simulink model "CrCtl_Governor"  (R2016b)
settings: configuration reference "CodeGenConfigSet" (kept outside this file)
values from neighbouring files (symbols this model uses):
  ACC_ZERO = fi(0,Acc_m_s2)    [init_CrCtl_Governor.m]
  CrCtl_facAcc2TrqCor_C = Calibration.Parameter    [init_CrCtl_Governor.m]
  CrCtl_facDecl2TrqCor_C = Calibration.Parameter    [init_CrCtl_Governor.m]
  CrCtl_facPT11_C = Calibration.Parameter    [init_CrCtl_Governor.m]
  CrCtl_facPT12_C = Calibration.Parameter    [init_CrCtl_Governor.m]
  CrCtl_facPT13_C = Calibration.Parameter    [init_CrCtl_Governor.m]
  CrCtl_facRmpSlpHiAcc_C = Calibration.Parameter    [init_CrCtl_Governor.m]
  CrCtl_facRmpSlpHiDecl_C = Calibration.Parameter    [init_CrCtl_Governor.m]
  CrCtl_facSlpConstRmpDwn_C = Calibration.Parameter    [init_CrCtl_Governor.m]
  CrCtl_facSlpConstRmpUp_C = Calibration.Parameter    [init_CrCtl_Governor.m]
  CrCtl_facSlpRmp1Sus_C = Calibration.Parameter    [init_CrCtl_Governor.m]
  CrCtl_facSlpRmp2Sus_C = Calibration.Parameter    [init_CrCtl_Governor.m]
  CrCtl_facTipDwnCor_CUR = Calibration.Parameter    [init_CrCtl_Governor.m]
  CrCtl_facTipDwnCor_CURX = Calibration.Parameter    [init_CrCtl_Governor.m]
  CrCtl_facTipUpCor_CUR = Calibration.Parameter    [init_CrCtl_Governor.m]
  CrCtl_facTipUpCor_CURX = Calibration.Parameter    [init_CrCtl_Governor.m]
  CrCtl_facTrqIncrSlpConstRmp_C = Calibration.Parameter    [init_CrCtl_Governor.m]
  CrCtl_facTrqIncrTimeConstRmp_C = Calibration.Parameter    [init_CrCtl_Governor.m]
  CrCtl_facTrqRedSlpConstRmp_C = Calibration.Parameter    [init_CrCtl_Governor.m]
  CrCtl_facTrqRedTimeConstRmp_C = Calibration.Parameter    [init_CrCtl_Governor.m]
  CrCtl_facTrqStrtAcc_C = Calibration.Parameter    [init_CrCtl_Governor.m]
  CrCtl_KiAcc1IWin_C = Calibration.Parameter    [init_CrCtl_Governor.m]
  CrCtl_KiAcc2IWin_C = Calibration.Parameter    [init_CrCtl_Governor.m]
  CrCtl_KiAcc3IWin_C = Calibration.Parameter    [init_CrCtl_Governor.m]
  CrCtl_KiCruise1IWin_C = Calibration.Parameter    [init_CrCtl_Governor.m]
  CrCtl_KiCruise2IWin_C = Calibration.Parameter    [init_CrCtl_Governor.m]
  CrCtl_KiCruise3IWin_C = Calibration.Parameter    [init_CrCtl_Governor.m]
  CrCtl_KiDecl1IWin_C = Calibration.Parameter    [init_CrCtl_Governor.m]
  CrCtl_KiDecl2IWin_C = Calibration.Parameter    [init_CrCtl_Governor.m]
  CrCtl_KiDecl3IWin_C = Calibration.Parameter    [init_CrCtl_Governor.m]
  CrCtl_KiNegAcc1IWin_C = Calibration.Parameter    [init_CrCtl_Governor.m]
  CrCtl_KiNegAcc2IWin_C = Calibration.Parameter    [init_CrCtl_Governor.m]
  CrCtl_KiNegAcc3IWin_C = Calibration.Parameter    [init_CrCtl_Governor.m]
  CrCtl_KiNegCruise1IWin_C = Calibration.Parameter    [init_CrCtl_Governor.m]
  CrCtl_KiNegCruise2IWin_C = Calibration.Parameter    [init_CrCtl_Governor.m]
  CrCtl_KiNegCruise3IWin_C = Calibration.Parameter    [init_CrCtl_Governor.m]
  CrCtl_KiNegDecl1IWin_C = Calibration.Parameter    [init_CrCtl_Governor.m]
  CrCtl_KiNegDecl2IWin_C = Calibration.Parameter    [init_CrCtl_Governor.m]
  CrCtl_KiNegDecl3IWin_C = Calibration.Parameter    [init_CrCtl_Governor.m]
  CrCtl_KiNegRes1IWin_C = Calibration.Parameter    [init_CrCtl_Governor.m]
  CrCtl_KiNegRes2IWin_C = Calibration.Parameter    [init_CrCtl_Governor.m]
  CrCtl_KiNegRes3IWin_C = Calibration.Parameter    [init_CrCtl_Governor.m]
  CrCtl_KiNegResCruise1IWin_C = Calibration.Parameter    [init_CrCtl_Governor.m]
  CrCtl_KiNegResCruise2IWin_C = Calibration.Parameter    [init_CrCtl_Governor.m]
  CrCtl_KiNegResCruise3IWin_C = Calibration.Parameter    [init_CrCtl_Governor.m]
  CrCtl_KiPosAcc1IWin_C = Calibration.Parameter    [init_CrCtl_Governor.m]
  CrCtl_KiPosAcc2IWin_C = Calibration.Parameter    [init_CrCtl_Governor.m]
  CrCtl_KiPosAcc3IWin_C = Calibration.Parameter    [init_CrCtl_Governor.m]
  CrCtl_KiPosCruise1IWin_C = Calibration.Parameter    [init_CrCtl_Governor.m]
  CrCtl_KiPosCruise2IWin_C = Calibration.Parameter    [init_CrCtl_Governor.m]
  CrCtl_KiPosCruise3IWin_C = Calibration.Parameter    [init_CrCtl_Governor.m]
  CrCtl_KiPosDecl1IWin_C = Calibration.Parameter    [init_CrCtl_Governor.m]
  CrCtl_KiPosDecl2IWin_C = Calibration.Parameter    [init_CrCtl_Governor.m]
  CrCtl_KiPosDecl3IWin_C = Calibration.Parameter    [init_CrCtl_Governor.m]
  CrCtl_KiPosRes1IWin_C = Calibration.Parameter    [init_CrCtl_Governor.m]
  CrCtl_KiPosRes3IWin_C = Calibration.Parameter    [init_CrCtl_Governor.m]
  CrCtl_KiPosResCruise1IWin_C = Calibration.Parameter    [init_CrCtl_Governor.m]
  CrCtl_KiPosResCruise2IWin_C = Calibration.Parameter    [init_CrCtl_Governor.m]
  CrCtl_KiPosResCruise3IWin_C = Calibration.Parameter    [init_CrCtl_Governor.m]
  CrCtl_KiRes1IWin_C = Calibration.Parameter    [init_CrCtl_Governor.m]
  CrCtl_KiRes2IWin_C = Calibration.Parameter    [init_CrCtl_Governor.m]
  CrCtl_KiRes3IWin_C = Calibration.Parameter    [init_CrCtl_Governor.m]
  CrCtl_KiResCruise1IWin_C = Calibration.Parameter    [init_CrCtl_Governor.m]
  CrCtl_KiResCruise2IWin_C = Calibration.Parameter    [init_CrCtl_Governor.m]
  CrCtl_KiResCruise3IWin_C = Calibration.Parameter    [init_CrCtl_Governor.m]
  CrCtl_KpAcc1PWin_C = Calibration.Parameter    [init_CrCtl_Governor.m]
  CrCtl_KpAcc2PWin_C = Calibration.Parameter    [init_CrCtl_Governor.m]
  CrCtl_KpAcc3PWin_C = Calibration.Parameter    [init_CrCtl_Governor.m]
  CrCtl_KpCruise1PWin_C = Calibration.Parameter    [init_CrCtl_Governor.m]
  CrCtl_KpCruise2PWin_C = Calibration.Parameter    [init_CrCtl_Governor.m]
  CrCtl_KpCruise3PWin_C = Calibration.Parameter    [init_CrCtl_Governor.m]
  CrCtl_KpDecl1PWin_C = Calibration.Parameter    [init_CrCtl_Governor.m]
  CrCtl_KpDecl2PWin_C = Calibration.Parameter    [init_CrCtl_Governor.m]
  CrCtl_KpDecl3PWin_C = Calibration.Parameter    [init_CrCtl_Governor.m]
  CrCtl_KpNegAcc1PWin_C = Calibration.Parameter    [init_CrCtl_Governor.m]
  CrCtl_KpNegAcc2PWin_C = Calibration.Parameter    [init_CrCtl_Governor.m]
  CrCtl_KpNegAcc3PWin_C = Calibration.Parameter    [init_CrCtl_Governor.m]
  CrCtl_KpNegCruise1PWin_C = Calibration.Parameter    [init_CrCtl_Governor.m]
  CrCtl_KpNegCruise2PWin_C = Calibration.Parameter    [init_CrCtl_Governor.m]
  CrCtl_KpNegCruise3PWin_C = Calibration.Parameter    [init_CrCtl_Governor.m]
  CrCtl_KpNegDecl1PWin_C = Calibration.Parameter    [init_CrCtl_Governor.m]
  CrCtl_KpNegDecl2PWin_C = Calibration.Parameter    [init_CrCtl_Governor.m]
  CrCtl_KpNegDecl3PWin_C = Calibration.Parameter    [init_CrCtl_Governor.m]
  CrCtl_KpNegRes1PWin_C = Calibration.Parameter    [init_CrCtl_Governor.m]
  CrCtl_KpNegRes2PWin_C = Calibration.Parameter    [init_CrCtl_Governor.m]
  CrCtl_KpNegRes3PWin_C = Calibration.Parameter    [init_CrCtl_Governor.m]
  CrCtl_KpNegResCruise1PWin_C = Calibration.Parameter    [init_CrCtl_Governor.m]
  CrCtl_KpNegResCruise2PWin_C = Calibration.Parameter    [init_CrCtl_Governor.m]
  CrCtl_KpNegResCruise3PWin_C = Calibration.Parameter    [init_CrCtl_Governor.m]
  CrCtl_KpPosAcc1PWin_C = Calibration.Parameter    [init_CrCtl_Governor.m]
  CrCtl_KpPosAcc2PWin_C = Calibration.Parameter    [init_CrCtl_Governor.m]
  CrCtl_KpPosAcc3PWin_C = Calibration.Parameter    [init_CrCtl_Governor.m]
  CrCtl_KpPosCruise1PWin_C = Calibration.Parameter    [init_CrCtl_Governor.m]
  CrCtl_KpPosCruise2PWin_C = Calibration.Parameter    [init_CrCtl_Governor.m]
  CrCtl_KpPosCruise3PWin_C = Calibration.Parameter    [init_CrCtl_Governor.m]
  CrCtl_KpPosDecl1PWin_C = Calibration.Parameter    [init_CrCtl_Governor.m]
  CrCtl_KpPosDecl2PWin_C = Calibration.Parameter    [init_CrCtl_Governor.m]
  CrCtl_KpPosDecl3PWin_C = Calibration.Parameter    [init_CrCtl_Governor.m]
  CrCtl_KpPosRes1PWin_C = Calibration.Parameter    [init_CrCtl_Governor.m]
  CrCtl_KpPosRes2PWin_C = Calibration.Parameter    [init_CrCtl_Governor.m]
  CrCtl_KpPosRes3PWin_C = Calibration.Parameter    [init_CrCtl_Governor.m]
  CrCtl_KpPosResCruise1PWin_C = Calibration.Parameter    [init_CrCtl_Governor.m]
  CrCtl_KpPosResCruise2PWin_C = Calibration.Parameter    [init_CrCtl_Governor.m]
  CrCtl_KpPosResCruise3PWin_C = Calibration.Parameter    [init_CrCtl_Governor.m]
  CrCtl_KpRes1PWin_C = Calibration.Parameter    [init_CrCtl_Governor.m]
  CrCtl_KpRes2PWin_C = Calibration.Parameter    [init_CrCtl_Governor.m]
  CrCtl_KpRes3PWin_C = Calibration.Parameter    [init_CrCtl_Governor.m]
  CrCtl_KpResCruise1PWin_C = Calibration.Parameter    [init_CrCtl_Governor.m]
  CrCtl_KpResCruise2PWin_C = Calibration.Parameter    [init_CrCtl_Governor.m]
  CrCtl_KpResCruise3PWin_C = Calibration.Parameter    [init_CrCtl_Governor.m]
  CrCtl_numParSelThres1_C = Calibration.Parameter    [init_CrCtl_Governor.m]
  CrCtl_numParSelThres2_C = Calibration.Parameter    [init_CrCtl_Governor.m]
  CrCtl_swtBrkMode_C = Calibration.Parameter    [init_CrCtl_Governor.m]
  CrCtl_swtILimWithP_C = Calibration.Parameter    [init_CrCtl_Governor.m]
  CrCtl_swtOvrRdeFrzInteg_C = Calibration.Parameter    [init_CrCtl_Governor.m]
  CrCtl_swtParSelHysBrk_C = Calibration.Parameter    [init_CrCtl_Governor.m]
  CrCtl_swtPT1EngBrk_C = Calibration.Parameter    [init_CrCtl_Governor.m]
  CrCtl_swtSusRmpInit_C = Calibration.Parameter    [init_CrCtl_Governor.m]
  CrCtl_swtSusRmpStp_C = Calibration.Parameter    [init_CrCtl_Governor.m]
  CrCtl_swtTipUpDwnGvnrStrtVal_C = Calibration.Parameter    [init_CrCtl_Governor.m]
  ... (+88 more)
undefined symbols (not defined in the file or in its folder): CrCtl_Governor_DT, CrCtl_stLck_conv, CrCtl_stOpFunc_conv, CrCtl_stShOff_conv, CrCtl_stSub_conv, CrCtl_stSuspRamp_conv, CruiseCtl_State_conv, EBrk_stPreSelMode_conv, WESDem_State_conv
libraries: CXLib x126, simulink x25
(part 5 of 6)

== system CrCtl_Governor/Resume From Below/CRCTL_SUBRMP/Governor ==
  CrCtl_trqLimAct : Inport
  CrCtl_trqMin : Inport  Port=2
  CrCtl_stGearRng_mp : Inport  Port=3
  CrCtl_vDesAct : Inport  Port=4
  stvHysEngBrkReq : Inport  Port=5
  GlbDa_vXFlt : Inport  Port=6
  stCrCtlOn : Inport  Port=7
  In1 : Inport  Port=8
  In2 : Inport  Port=9
  Enable : EnablePort
  Add1 : Sum  Inputs=+-
  Add2 : Sum  OutDataTypeStr=Trq_Nm
  Add3 : Sum  OutDataTypeStr=Trq_Nm
  Constant : Constant  Value=CrCtl_swtILimWithP_C
  Constant1 : Constant  Value=CrCtl_Governor_DT
  Constant2 : Constant  Value=1000  OutDataTypeStr=Inherit: Inherit via back propagation
  CrCtl_ARW : Subsystem
  I_S16 : CXLib/I_S16
  PT1 Filtered Torque : Subsystem
  P_S16 : CXLib/P_S16
  Parameter Selection for Ki : Subsystem
  Parameter Selection for Kp : Subsystem
  Product : Product  OutDataTypeStr=uint32
  Saturation_S16 : CXLib/Saturation_S16
  Switch : Switch  Criteria=u2 ~= 0
  Terminator : Terminator
  Unit Delay : UnitDelay  SampleTime=-1
  Unit Delay1 : UnitDelay  SampleTime=-1
  CrCtl_trqReq : Outport
  CrCtl_trqIWinOld_mp : Outport  Port=2  OutDataTypeStr=Trq_Nm
  CrCtl_trqReqPWin_mp : Outport  Port=3
  wires:
  CrCtl_vDesAct/1 -> Add1/1
  GlbDa_vXFlt/1 -> Add1/2
  Add1/1 -> PT1 Filtered Torque/2(vDiffCrCtl), I_S16/1, P_S16/1
  Add2/1 -> Add3/1
  PT1 Filtered Torque/1(CrCtl_trqDesvHys) -> Add3/2
  Add3/1 -> Saturation_S16/1
  CrCtl_trqMin/1 -> CrCtl_ARW/2(CrCtl_trqMin), Saturation_S16/2
  CrCtl_trqLimAct/1 -> CrCtl_ARW/3(CrCtl_trqLimAct), Saturation_S16/3
  Saturation_S16/2 -> Terminator/1
  Saturation_S16/1 -> CrCtl_trqReq/1
  Switch/1 -> Add2/2, CrCtl_trqIWinOld_mp/1, CrCtl_ARW/5(CrCtl_trqReqIWin_mp)
  Constant/1 -> CrCtl_ARW/1(CrCtl_swtILimWithP_C)
  stvHysEngBrkReq/1 -> PT1 Filtered Torque/1(stvHysEngBrkReq)
  CrCtl_stGearRng_mp/1 -> Parameter Selection for Kp/1(CrCtl_stGearRng_mp), Parameter Selection for Ki/1(CrCtl_stGearRng_mp), PT1 Filtered Torque/3(CrCtl_stGearRng_mp)
  stCrCtlOn/1 -> PT1 Filtered Torque/4(stCrCtlOn)
  Parameter Selection for Kp/1(Out1) -> P_S16/2
  Parameter Selection for Kp/2(Out2) -> P_S16/3
  Parameter Selection for Kp/3(Out3) -> P_S16/4
  Parameter Selection for Kp/4(Out4) -> P_S16/5
  Parameter Selection for Kp/5(Out5) -> P_S16/6
  Parameter Selection for Ki/1(Out1) -> I_S16/3
  Parameter Selection for Ki/2(Out2) -> I_S16/4
  Parameter Selection for Ki/3(Out3) -> I_S16/5
  Parameter Selection for Ki/4(Out4) -> I_S16/6
  Parameter Selection for Ki/5(Out5) -> I_S16/7
  CrCtl_ARW/2(Limit) -> Unit Delay1/1
  CrCtl_ARW/1(CrCtl_stInit_mp) -> Unit Delay/1
  Product/1 -> I_S16/2
  Constant2/1 -> Product/2
  Constant1/1 -> Product/1
  P_S16/1 -> CrCtl_trqReqPWin_mp/1, CrCtl_ARW/4(CrCtl_trqReqPWin_mp), Add2/1
  In1/1 -> I_S16/8
  In2/1 -> I_S16/9
  I_S16/1 -> Switch/3
  Unit Delay/1 -> Switch/2
  Unit Delay1/1 -> Switch/1

== system CrCtl_Governor/Resume From Below/CRCTL_SUBSTRTVAL/Parameter Selection for Kp ==
  CrCtl_stGearRng_mp : Inport
  Constant1 : Constant  Value=CrCtl_KpRes2PWin_C
  Constant10 : Constant  Value=CrCtl_WinPosRes1PWin_C
  Constant11 : Constant  Value=CrCtl_WinPosRes2PWin_C
  Constant12 : Constant  Value=CrCtl_WinPosRes3PWin_C
  Constant13 : Constant  Value=CrCtl_WinNegRes1PWin_C
  Constant14 : Constant  Value=CrCtl_WinNegRes2PWin_C
  Constant15 : Constant  Value=CrCtl_WinNegRes3PWin_C
  Constant2 : Constant  Value=CrCtl_KpRes3PWin_C
  Constant3 : Constant  Value=CrCtl_KpPosRes1PWin_C
  Constant4 : Constant  Value=CrCtl_KpRes1PWin_C
  Constant5 : Constant  Value=CrCtl_KpPosRes2PWin_C
  Constant6 : Constant  Value=CrCtl_KpPosRes3PWin_C
  Constant7 : Constant  Value=CrCtl_KpNegRes1PWin_C
  Constant8 : Constant  Value=CrCtl_KpNegRes2PWin_C
  Constant9 : Constant  Value=CrCtl_KpNegRes3PWin_C
  Multiport Switch{,1..4} (5 alike) : MultiPortSwitch
  Out1 : Outport
  Out2 : Outport  Port=2
  Out3 : Outport  Port=3
  Out4 : Outport  Port=4
  Out5 : Outport  Port=5
  wires:
  CrCtl_stGearRng_mp/1 -> Multiport Switch4/1, Multiport Switch3/1, Multiport Switch2/1, Multiport Switch1/1, Multiport Switch/1
  Constant4/1 -> Multiport Switch/2
  Constant1/1 -> Multiport Switch/3
  Constant2/1 -> Multiport Switch/4
  Multiport Switch/1 -> Out1/1
  Constant3/1 -> Multiport Switch1/2
  Constant6/1 -> Multiport Switch1/4
  Constant5/1 -> Multiport Switch1/3
  Multiport Switch1/1 -> Out2/1
  Constant7/1 -> Multiport Switch2/2
  Constant9/1 -> Multiport Switch2/4
  Constant8/1 -> Multiport Switch2/3
  Constant10/1 -> Multiport Switch3/2
  Constant12/1 -> Multiport Switch3/4
  Constant11/1 -> Multiport Switch3/3
  Constant13/1 -> Multiport Switch4/2
  Constant15/1 -> Multiport Switch4/4
  Constant14/1 -> Multiport Switch4/3
  Multiport Switch2/1 -> Out3/1
  Multiport Switch3/1 -> Out4/1
  Multiport Switch4/1 -> Out5/1

== system CrCtl_Governor/Tip Down State/CRCTL_SUBCALCSET /Parameter Selection for Kp ==
  CrCtl_stGearRng_mp : Inport
  Constant1 : Constant  Value=CrCtl_KpDecl2PWin_C
  Constant10 : Constant  Value=CrCtl_WinPosDecl1PWin_C
  Constant11 : Constant  Value=CrCtl_WinPosDecl2PWin_C
  Constant12 : Constant  Value=CrCtl_WinPosDecl3PWin_C
  Constant13 : Constant  Value=CrCtl_WinNegDecl1PWin_C
  Constant14 : Constant  Value=CrCtl_WinNegDecl2PWin_C
  Constant15 : Constant  Value=CrCtl_WinNegDecl3PWin_C
  Constant2 : Constant  Value=CrCtl_KpDecl3PWin_C
  Constant3 : Constant  Value=CrCtl_KpPosDecl1PWin_C
  Constant4 : Constant  Value=CrCtl_KpDecl1PWin_C
  Constant5 : Constant  Value=CrCtl_KpPosDecl2PWin_C
  Constant6 : Constant  Value=CrCtl_KpPosDecl3PWin_C
  Constant7 : Constant  Value=CrCtl_KpNegDecl1PWin_C
  Constant8 : Constant  Value=CrCtl_KpNegDecl2PWin_C
  Constant9 : Constant  Value=CrCtl_KpNegDecl3PWin_C
  Multiport Switch{,1..4} (5 alike) : MultiPortSwitch
  Out1 : Outport
  Out2 : Outport  Port=2
  Out3 : Outport  Port=3
  Out4 : Outport  Port=4
  Out5 : Outport  Port=5
  wires:
  CrCtl_stGearRng_mp/1 -> Multiport Switch4/1, Multiport Switch3/1, Multiport Switch2/1, Multiport Switch1/1, Multiport Switch/1
  Constant4/1 -> Multiport Switch/2
  Constant1/1 -> Multiport Switch/3
  Constant2/1 -> Multiport Switch/4
  Multiport Switch/1 -> Out1/1
  Constant3/1 -> Multiport Switch1/2
  Constant6/1 -> Multiport Switch1/4
  Constant5/1 -> Multiport Switch1/3
  Multiport Switch1/1 -> Out2/1
  Constant7/1 -> Multiport Switch2/2
  Constant9/1 -> Multiport Switch2/4
  Constant8/1 -> Multiport Switch2/3
  Constant10/1 -> Multiport Switch3/2
  Constant12/1 -> Multiport Switch3/4
  Constant11/1 -> Multiport Switch3/3
  Constant13/1 -> Multiport Switch4/2
  Constant15/1 -> Multiport Switch4/4
  Constant14/1 -> Multiport Switch4/3
  Multiport Switch2/1 -> Out3/1
  Multiport Switch3/1 -> Out4/1
  Multiport Switch4/1 -> Out5/1

== system CrCtl_Governor/Tip Up State/Subsystem/Parameter Selection for Kp ==
  CrCtl_stGearRng_mp : Inport
  Constant1 : Constant  Value=CrCtl_KpAcc2PWin_C
  Constant10 : Constant  Value=CrCtl_WinPosAcc1PWin_C
  Constant11 : Constant  Value=CrCtl_WinPosAcc2PWin_C
  Constant12 : Constant  Value=CrCtl_WinPosAcc3PWin_C
  Constant13 : Constant  Value=CrCtl_WinNegAcc1PWin_C
  Constant14 : Constant  Value=CrCtl_WinNegAcc2PWin_C
  Constant15 : Constant  Value=CrCtl_WinNegAcc3PWin_C
  Constant2 : Constant  Value=CrCtl_KpAcc3PWin_C
  Constant3 : Constant  Value=CrCtl_KpPosAcc1PWin_C
  Constant4 : Constant  Value=CrCtl_KpAcc1PWin_C
  Constant5 : Constant  Value=CrCtl_KpPosAcc2PWin_C
  Constant6 : Constant  Value=CrCtl_KpPosAcc3PWin_C
  Constant7 : Constant  Value=CrCtl_KpNegAcc1PWin_C
  Constant8 : Constant  Value=CrCtl_KpNegAcc2PWin_C
  Constant9 : Constant  Value=CrCtl_KpNegAcc3PWin_C
  Multiport Switch{,1..4} (5 alike) : MultiPortSwitch
  Out1 : Outport
  Out2 : Outport  Port=2
  Out3 : Outport  Port=3
  Out4 : Outport  Port=4
  Out5 : Outport  Port=5
  wires:
  CrCtl_stGearRng_mp/1 -> Multiport Switch4/1, Multiport Switch3/1, Multiport Switch2/1, Multiport Switch1/1, Multiport Switch/1
  Constant4/1 -> Multiport Switch/2
  Constant1/1 -> Multiport Switch/3
  Constant2/1 -> Multiport Switch/4
  Multiport Switch/1 -> Out1/1
  Constant3/1 -> Multiport Switch1/2
  Constant6/1 -> Multiport Switch1/4
  Constant5/1 -> Multiport Switch1/3
  Multiport Switch1/1 -> Out2/1
  Constant7/1 -> Multiport Switch2/2
  Constant9/1 -> Multiport Switch2/4
  Constant8/1 -> Multiport Switch2/3
  Constant10/1 -> Multiport Switch3/2
  Constant12/1 -> Multiport Switch3/4
  Constant11/1 -> Multiport Switch3/3
  Constant13/1 -> Multiport Switch4/2
  Constant15/1 -> Multiport Switch4/4
  Constant14/1 -> Multiport Switch4/3
  Multiport Switch2/1 -> Out3/1
  Multiport Switch3/1 -> Out4/1
  Multiport Switch4/1 -> Out5/1

== system CrCtl_Governor/Acceleration State/CRCTL_SUBRMP/CrCtl_Suspend/Subsystem ==
  PT_trqWhlMinEng : Inport
  CrCtl_trqReqOld : Inport  Port=2
  CrCtl_stSuspAct : Inport  Port=3
  Enable : EnablePort
  Constant5 : Constant  Value=CrCtl_swtSusRmpStp_C
  Constant7 : Constant  Value=CrCtl_facSlpRmp1Sus_C
  Constant8 : Constant  Value=CrCtl_Governor_DT
  RAMP_S16 : CXLib/RAMP_S16
  Relational Operator : RelationalOperator  Operator=~=  OutDataTypeStr=boolean  RndMeth=Simplest
  Switch3 : Switch  Criteria=u2 ~= 0
  s2dt : CXLib/s2dt
  Out : Outport
  Out1 : Outport  Port=2
  wires:
  Constant7/1 -> s2dt/1
  Constant8/1 -> s2dt/2
  s2dt/1 -> RAMP_S16/3, RAMP_S16/2
  CrCtl_stSuspAct/1 -> RAMP_S16/4
  PT_trqWhlMinEng/1 -> Relational Operator/1, Switch3/1, RAMP_S16/1
  Relational Operator/1 -> Out/1
  CrCtl_trqReqOld/1 -> RAMP_S16/5
  Constant5/1 -> Switch3/2
  Switch3/1 -> Relational Operator/2, Out1/1
  RAMP_S16/1 -> Switch3/3

== system CrCtl_Governor/Acceleration State/CRCTL_SUBRMP/CrCtl_Suspend/Subsystem1 ==
  PT_trqWhlMinEng : Inport
  CrCtl_trqReqOld : Inport  Port=2
  AccPed_trqDes : Inport  Port=3
  CrCtl_trqLimAct : Inport  Port=4
  In1 : Inport  Port=5
  In2 : Inport  Port=6
  In3 : Inport  Port=7
  Enable : EnablePort
  Constant10 : Constant  Value=CrCtl_Governor_DT
  Constant6 : Constant  Value=CrCtl_swtSusRmpInit_C
  Constant9 : Constant  Value=CrCtl_facSlpRmp2Sus_C
  MinMax : MinMax  Function=max  Inputs=2
  MinMax1 : MinMax  Function=max  Inputs=2
  RAMP_S1 : CXLib/RAMP_S16
  Relational Operator1 : RelationalOperator  Operator=~=  OutDataTypeStr=boolean  RndMeth=Simplest
  Relational Operator2 : RelationalOperator  Operator=<  OutDataTypeStr=boolean  RndMeth=Simplest
  Relational Operator3 : RelationalOperator  Operator=<  OutDataTypeStr=boolean  RndMeth=Simplest
  Relational Operator4 : RelationalOperator  Operator=<  OutDataTypeStr=boolean  RndMeth=Simplest
  Switch{1..4,6} (5 alike) : Switch  Criteria=u2 ~= 0
  s2dt1 : CXLib/s2dt
  Out1 : Outport
  Out2 : Outport  Port=2
  wires:
  Constant9/1 -> s2dt1/1
  Constant10/1 -> s2dt1/2
  s2dt1/1 -> RAMP_S1/3, RAMP_S1/2
  CrCtl_trqReqOld/1 -> RAMP_S1/1, Relational Operator4/1, Switch6/1, MinMax/1, Relational Operator1/2, Switch2/1, Relational Operator3/1
  Constant6/1 -> Switch3/2
  MinMax/1 -> MinMax1/1
  MinMax1/1 -> Switch4/1, Relational Operator2/1
  CrCtl_trqLimAct/1 -> Switch4/3, Relational Operator2/2
  Relational Operator2/1 -> Switch4/2
  Switch4/1 -> Switch3/1
  AccPed_trqDes/1 -> Relational Operator3/2, MinMax1/2
  PT_trqWhlMinEng/1 -> Switch1/1, Relational Operator4/2, MinMax/2
  Relational Operator4/1 -> Switch1/2
  Switch3/1 -> Switch1/3
  Switch1/1 -> RAMP_S1/5
  In3/1 -> RAMP_S1/4
  In1/1 -> Switch6/2
  In2/1 -> Switch6/3
  Switch6/1 -> Switch3/3
  Relational Operator3/1 -> Switch2/2
  RAMP_S1/1 -> Switch2/3
  Switch2/1 -> Out2/1, Relational Operator1/1
  Relational Operator1/1 -> Out1/1

== system CrCtl_Governor/Acceleration State/CRCTL_SUBRMP/Governor/CrCtl_ARW ==
  CrCtl_swtILimWithP_C : Inport
  CrCtl_trqMin : Inport  Port=2
  CrCtl_trqLimAct : Inport  Port=3
  CrCtl_trqReqPWin_mp : Inport  Port=4
  CrCtl_trqReqIWin_mp : Inport  Port=5
  Add : Sum  Inputs=+-  OutDataTypeStr=Trq_Nm
  Add1 : Sum  Inputs=+-  OutDataTypeStr=Trq_Nm
  Relational Operator : RelationalOperator  Operator=<  OutDataTypeStr=boolean  RndMeth=Simplest
  Relational Operator1 : RelationalOperator  Operator=>  OutDataTypeStr=boolean  RndMeth=Simplest
  Saturation_S1 : CXLib/Saturation_S16
  Saturation_S16 : CXLib/Saturation_S16
  Switch{,1..3} (4 alike) : Switch  Criteria=u2 ~= 0
  CrCtl_stInit_mp : Outport
  Limit : Outport  Port=2
  wires:
  CrCtl_trqMin/1 -> Switch2/3, Relational Operator/2, Add/1, Saturation_S16/2
  CrCtl_trqLimAct/1 -> Switch3/3, Relational Operator1/2, Add1/1, Saturation_S16/3
  CrCtl_trqReqIWin_mp/1 -> Relational Operator1/1, Relational Operator/1, Saturation_S1/1, Saturation_S16/1
  CrCtl_swtILimWithP_C/1 -> Switch1/2, Switch/2
  Switch/1 -> CrCtl_stInit_mp/1
  Saturation_S16/2 -> Switch/3
  CrCtl_trqReqPWin_mp/1 -> Add1/2, Add/2
  Saturation_S1/2 -> Switch/1
  Saturation_S1/1 -> Switch1/1
  Saturation_S16/1 -> Switch1/3
  Switch1/1 -> Limit/1
  Switch2/1 -> Saturation_S1/2
  Switch3/1 -> Saturation_S1/3
  Add/1 -> Switch2/1
  Add1/1 -> Switch3/1
  Relational Operator/1 -> Switch2/2
  Relational Operator1/1 -> Switch3/2

== system CrCtl_Governor/Acceleration State/CRCTL_SUBRMP/Governor/PT1 Filtered Torque ==
  stvHysEngBrkReq : Inport
  vDiffCrCtl : Inport  Port=2
  CrCtl_stGearRng_mp : Inport  Port=3
  stCrCtlOn : Inport  Port=4
  Add : Sum  Inputs=+-
  Constant : Constant
  Constant1 : Constant  Value=CrCtl_swtPT1EngBrk_C
  Constant2 : Constant  Value=CrCtl_vEngBrkOffChkOfs_C
  Constant3 : Constant  Value=CrCtl_vHysEngBrkMode_C
  Constant4 : Constant  Value=0.0  OutDataTypeStr=Inherit: Inherit via back propagation
  Constant5 : Constant  Value=0  OutDataTypeStr=VehSpeed_km_h
  Logical Operator : Logic  Operator=NOT  AllPortsSameDT=off  OutDataTypeStr=boolean
  Logical Operator1 : Logic  Operator=OR  AllPortsSameDT=off  OutDataTypeStr=boolean
  PT1_S16 : CXLib/PT1_S16
  Parameter selection of PT1 : Subsystem
  Product : Product  OutDataTypeStr=Trq_Nm
  Relational Operator : RelationalOperator  Operator===  OutDataTypeStr=boolean  RndMeth=Simplest
  Switch : Switch  Criteria=u2 ~= 0
  Switch1 : Switch  Criteria=u2 ~= 0
  Switch2 : Switch  Criteria=u2 ~= 0
  CrCtl_trqDesvHys : Outport
  wires:
  Constant1/1 -> Relational Operator/1
  Constant/1 -> Relational Operator/2
  stvHysEngBrkReq/1 -> Logical Operator/1
  Relational Operator/1 -> Logical Operator1/1
  Logical Operator/1 -> Logical Operator1/2
  Constant2/1 -> Add/1
  Constant3/1 -> Add/2
  Logical Operator1/1 -> Switch1/2, Switch/2
  Add/1 -> Switch/3
  vDiffCrCtl/1 -> Switch/1
  CrCtl_stGearRng_mp/1 -> Parameter selection of PT1/1(CrCtl_stGearRng_mp)
  Parameter selection of PT1/1(Out1) -> PT1_S16/1
  Product/1 -> PT1_S16/2
  Parameter selection of PT1/2(Out2) -> Product/1
  PT1_S16/1 -> Switch1/1
  Constant4/1 -> Switch1/3
  Switch1/1 -> CrCtl_trqDesvHys/1  "CrCtl_trqPT1_mp"
  stCrCtlOn/1 -> Switch2/2
  Switch/1 -> Switch2/1
  Constant5/1 -> Switch2/3
  Switch2/1 -> Product/2

== system CrCtl_Governor/Acceleration State/CRCTL_SUBRMP/Governor/Parameter Selection for Ki ==
  CrCtl_stGearRng_mp : Inport
  Constant1 : Constant  Value=CrCtl_KiAcc2IWin_C
  Constant10 : Constant  Value=CrCtl_WinPosAcc1IWin_C
  Constant11 : Constant  Value=CrCtl_WinPosAcc2IWin_C
  Constant12 : Constant  Value=CrCtl_WinPosAcc3IWin_C
  Constant13 : Constant  Value=CrCtl_WinNegAcc1IWin_C
  Constant14 : Constant  Value=CrCtl_WinNegAcc2IWin_C
  Constant15 : Constant  Value=CrCtl_WinNegAcc3IWin_C
  Constant2 : Constant  Value=CrCtl_KiAcc3IWin_C
  Constant3 : Constant  Value=CrCtl_KiPosAcc1IWin_C
  Constant4 : Constant  Value=CrCtl_KiAcc1IWin_C
  Constant5 : Constant  Value=CrCtl_KiPosAcc2IWin_C
  Constant6 : Constant  Value=CrCtl_KiPosAcc3IWin_C
  Constant7 : Constant  Value=CrCtl_KiNegAcc1IWin_C
  Constant8 : Constant  Value=CrCtl_KiNegAcc2IWin_C
  Constant9 : Constant  Value=CrCtl_KiNegAcc3IWin_C
  Multiport Switch{,1..4} (5 alike) : MultiPortSwitch
  Out1 : Outport
  Out2 : Outport  Port=2
  Out3 : Outport  Port=3
  Out4 : Outport  Port=4
  Out5 : Outport  Port=5
  wires:
  Multiport Switch4/1 -> Out5/1
  Multiport Switch3/1 -> Out4/1
  Multiport Switch2/1 -> Out3/1
  Constant14/1 -> Multiport Switch4/3
  Constant15/1 -> Multiport Switch4/4
  Constant13/1 -> Multiport Switch4/2
  Constant11/1 -> Multiport Switch3/3
  Constant12/1 -> Multiport Switch3/4
  Constant10/1 -> Multiport Switch3/2
  Constant8/1 -> Multiport Switch2/3
  Constant9/1 -> Multiport Switch2/4
  Constant7/1 -> Multiport Switch2/2
  Multiport Switch1/1 -> Out2/1
  Constant5/1 -> Multiport Switch1/3
  Constant6/1 -> Multiport Switch1/4
  Constant3/1 -> Multiport Switch1/2
  Multiport Switch/1 -> Out1/1
  Constant2/1 -> Multiport Switch/4
  Constant1/1 -> Multiport Switch/3
  Constant4/1 -> Multiport Switch/2
  CrCtl_stGearRng_mp/1 -> Multiport Switch/1, Multiport Switch1/1, Multiport Switch2/1, Multiport Switch3/1, Multiport Switch4/1

== system CrCtl_Governor/Acceleration State/CRCTL_SUBRMP/Governor/Parameter Selection for Kp ==
  CrCtl_stGearRng_mp : Inport
  Constant1 : Constant  Value=CrCtl_KpAcc2PWin_C
  Constant10 : Constant  Value=CrCtl_WinPosAcc1PWin_C
  Constant11 : Constant  Value=CrCtl_WinPosAcc2PWin_C
  Constant12 : Constant  Value=CrCtl_WinPosAcc3PWin_C
  Constant13 : Constant  Value=CrCtl_WinNegAcc1PWin_C
  Constant14 : Constant  Value=CrCtl_WinNegAcc2PWin_C
  Constant15 : Constant  Value=CrCtl_WinNegAcc3PWin_C
  Constant2 : Constant  Value=CrCtl_KpAcc3PWin_C
  Constant3 : Constant  Value=CrCtl_KpPosAcc1PWin_C
  Constant4 : Constant  Value=CrCtl_KpAcc1PWin_C
  Constant5 : Constant  Value=CrCtl_KpPosAcc2PWin_C
  Constant6 : Constant  Value=CrCtl_KpPosAcc3PWin_C
  Constant7 : Constant  Value=CrCtl_KpNegAcc1PWin_C
  Constant8 : Constant  Value=CrCtl_KpNegAcc2PWin_C
  Constant9 : Constant  Value=CrCtl_KpNegAcc3PWin_C
  Multiport Switch{,1..4} (5 alike) : MultiPortSwitch
  Out1 : Outport
  Out2 : Outport  Port=2
  Out3 : Outport  Port=3
  Out4 : Outport  Port=4
  Out5 : Outport  Port=5
  wires:
  CrCtl_stGearRng_mp/1 -> Multiport Switch4/1, Multiport Switch3/1, Multiport Switch2/1, Multiport Switch1/1, Multiport Switch/1
  Constant4/1 -> Multiport Switch/2
  Constant1/1 -> Multiport Switch/3
  Constant2/1 -> Multiport Switch/4
  Multiport Switch/1 -> Out1/1
  Constant3/1 -> Multiport Switch1/2
  Constant6/1 -> Multiport Switch1/4
  Constant5/1 -> Multiport Switch1/3
  Multiport Switch1/1 -> Out2/1
  Constant7/1 -> Multiport Switch2/2
  Constant9/1 -> Multiport Switch2/4
  Constant8/1 -> Multiport Switch2/3
  Constant10/1 -> Multiport Switch3/2
  Constant12/1 -> Multiport Switch3/4
  Constant11/1 -> Multiport Switch3/3
  Constant13/1 -> Multiport Switch4/2
  Constant15/1 -> Multiport Switch4/4
  Constant14/1 -> Multiport Switch4/3
  Multiport Switch2/1 -> Out3/1
  Multiport Switch3/1 -> Out4/1
  Multiport Switch4/1 -> Out5/1

== system CrCtl_Governor/Cruise State/CRCTL_SUBGVNR/CrCtl_Suspend/Subsystem ==
  PT_trqWhlMinEng : Inport
  CrCtl_trqReqOld : Inport  Port=2
  CrCtl_stSuspAct : Inport  Port=3
  Enable : EnablePort
  Constant5 : Constant  Value=CrCtl_swtSusRmpStp_C
  Constant7 : Constant  Value=CrCtl_facSlpRmp1Sus_C
  Constant8 : Constant  Value=CrCtl_Governor_DT
  RAMP_S16 : CXLib/RAMP_S16
  Relational Operator : RelationalOperator  Operator=~=  OutDataTypeStr=boolean  RndMeth=Simplest
  Switch3 : Switch  Criteria=u2 ~= 0
  s2dt : CXLib/s2dt
  Out : Outport
  Out1 : Outport  Port=2
  wires:
  Constant7/1 -> s2dt/1
  Constant8/1 -> s2dt/2
  s2dt/1 -> RAMP_S16/3, RAMP_S16/2
  CrCtl_stSuspAct/1 -> RAMP_S16/4
  PT_trqWhlMinEng/1 -> Relational Operator/1, Switch3/1, RAMP_S16/1
  Relational Operator/1 -> Out/1
  CrCtl_trqReqOld/1 -> RAMP_S16/5
  Constant5/1 -> Switch3/2
  Switch3/1 -> Relational Operator/2, Out1/1
  RAMP_S16/1 -> Switch3/3

== system CrCtl_Governor/Cruise State/CRCTL_SUBGVNR/CrCtl_Suspend/Subsystem1 ==
  PT_trqWhlMinEng : Inport
  CrCtl_trqReqOld : Inport  Port=2
  AccPed_trqDes : Inport  Port=3
  CrCtl_trqLimAct : Inport  Port=4
  In1 : Inport  Port=5
  In2 : Inport  Port=6
  In3 : Inport  Port=7
  Enable : EnablePort
  Constant10 : Constant  Value=CrCtl_Governor_DT
  Constant6 : Constant  Value=CrCtl_swtSusRmpInit_C
  Constant9 : Constant  Value=CrCtl_facSlpRmp2Sus_C
  MinMax : MinMax  Function=max  Inputs=2
  MinMax1 : MinMax  Function=max  Inputs=2
  RAMP_S1 : CXLib/RAMP_S16
  Relational Operator1 : RelationalOperator  Operator=~=  OutDataTypeStr=boolean  RndMeth=Simplest
  Relational Operator2 : RelationalOperator  Operator=<  OutDataTypeStr=boolean  RndMeth=Simplest
  Relational Operator3 : RelationalOperator  Operator=<  OutDataTypeStr=boolean  RndMeth=Simplest
  Relational Operator4 : RelationalOperator  Operator=<  OutDataTypeStr=boolean  RndMeth=Simplest
  Switch{1..4,6} (5 alike) : Switch  Criteria=u2 ~= 0
  s2dt1 : CXLib/s2dt
  Out1 : Outport
  Out2 : Outport  Port=2
  wires:
  Constant9/1 -> s2dt1/1
  Constant10/1 -> s2dt1/2
  s2dt1/1 -> RAMP_S1/3, RAMP_S1/2
  CrCtl_trqReqOld/1 -> RAMP_S1/1, Relational Operator4/1, Switch6/1, MinMax/1, Relational Operator1/2, Switch2/1, Relational Operator3/1
  Constant6/1 -> Switch3/2
  MinMax/1 -> MinMax1/1
  MinMax1/1 -> Switch4/1, Relational Operator2/1
  CrCtl_trqLimAct/1 -> Switch4/3, Relational Operator2/2
  Relational Operator2/1 -> Switch4/2
  Switch4/1 -> Switch3/1
  AccPed_trqDes/1 -> Relational Operator3/2, MinMax1/2
  PT_trqWhlMinEng/1 -> Switch1/1, Relational Operator4/2, MinMax/2
  Relational Operator4/1 -> Switch1/2
  Switch3/1 -> Switch1/3
  Switch1/1 -> RAMP_S1/5
  In3/1 -> RAMP_S1/4
  In1/1 -> Switch6/2
  In2/1 -> Switch6/3
  Switch6/1 -> Switch3/3
  Relational Operator3/1 -> Switch2/2
  RAMP_S1/1 -> Switch2/3
  Switch2/1 -> Out2/1, Relational Operator1/1
  Relational Operator1/1 -> Out1/1

== system CrCtl_Governor/Cruise State/CRCTL_SUBGVNR/Governor/CrCtl_ARW ==
  CrCtl_swtILimWithP_C : Inport
  CrCtl_trqMin : Inport  Port=2
  CrCtl_trqLimAct : Inport  Port=3
  CrCtl_trqReqPWin_mp : Inport  Port=4
  CrCtl_trqReqIWin_mp : Inport  Port=5
  Add : Sum  Inputs=+-  OutDataTypeStr=Trq_Nm
  Add1 : Sum  Inputs=+-  OutDataTypeStr=Trq_Nm
  Relational Operator : RelationalOperator  Operator=<  OutDataTypeStr=boolean  RndMeth=Simplest
  Relational Operator1 : RelationalOperator  Operator=>  OutDataTypeStr=boolean  RndMeth=Simplest
  Saturation_S1 : CXLib/Saturation_S16
  Saturation_S16 : CXLib/Saturation_S16
  Switch{,1..3} (4 alike) : Switch  Criteria=u2 ~= 0
  CrCtl_stInit_mp : Outport
  Limit : Outport  Port=2
  wires:
  CrCtl_trqMin/1 -> Switch2/3, Relational Operator/2, Add/1, Saturation_S16/2
  CrCtl_trqLimAct/1 -> Switch3/3, Relational Operator1/2, Add1/1, Saturation_S16/3
  CrCtl_trqReqIWin_mp/1 -> Relational Operator1/1, Relational Operator/1, Saturation_S1/1, Saturation_S16/1
  CrCtl_swtILimWithP_C/1 -> Switch1/2, Switch/2
  Switch/1 -> CrCtl_stInit_mp/1
  Saturation_S16/2 -> Switch/3
  CrCtl_trqReqPWin_mp/1 -> Add1/2, Add/2
  Saturation_S1/2 -> Switch/1
  Saturation_S1/1 -> Switch1/1
  Saturation_S16/1 -> Switch1/3
  Switch1/1 -> Limit/1
  Switch2/1 -> Saturation_S1/2
  Switch3/1 -> Saturation_S1/3
  Add/1 -> Switch2/1
  Add1/1 -> Switch3/1
  Relational Operator/1 -> Switch2/2
  Relational Operator1/1 -> Switch3/2

== system CrCtl_Governor/Cruise State/CRCTL_SUBGVNR/Governor/PT1 Filtered Torque ==
  stvHysEngBrkReq : Inport
  vDiffCrCtl : Inport  Port=2
  CrCtl_stGearRng_mp : Inport  Port=3
  stCrCtlOn : Inport  Port=4
  Add : Sum  Inputs=+-
  Constant : Constant  OutDataTypeStr=boolean
  Constant1 : Constant  Value=CrCtl_swtPT1EngBrk_C
  Constant2 : Constant  Value=CrCtl_vEngBrkOffChkOfs_C
  Constant3 : Constant  Value=CrCtl_vHysEngBrkMode_C
  Constant4 : Constant  Value=0.0  OutDataTypeStr=Inherit: Inherit via back propagation
  Constant5 : Constant  Value=0  OutDataTypeStr=VehSpeed_km_h
  Logical Operator : Logic  Operator=NOT  AllPortsSameDT=off  OutDataTypeStr=boolean
  Logical Operator1 : Logic  Operator=OR  AllPortsSameDT=off  OutDataTypeStr=boolean
  PT1_S16 : CXLib/PT1_S16
  Parameter selection of PT1 : Subsystem
  Product : Product  OutDataTypeStr=Trq_Nm
  Relational Operator : RelationalOperator  Operator===  OutDataTypeStr=boolean  RndMeth=Simplest
  Switch : Switch  Criteria=u2 ~= 0
  Switch1 : Switch  Criteria=u2 ~= 0
  Switch2 : Switch  Criteria=u2 ~= 0
  CrCtl_trqDesvHys : Outport
  wires:
  Constant1/1 -> Relational Operator/1
  Constant/1 -> Relational Operator/2
  stvHysEngBrkReq/1 -> Logical Operator/1
  Relational Operator/1 -> Logical Operator1/1
  Logical Operator/1 -> Logical Operator1/2
  Constant2/1 -> Add/1
  Constant3/1 -> Add/2
  Logical Operator1/1 -> Switch1/2, Switch/2
  Add/1 -> Switch/3
  vDiffCrCtl/1 -> Switch/1
  CrCtl_stGearRng_mp/1 -> Parameter selection of PT1/1(CrCtl_stGearRng_mp)
  Parameter selection of PT1/1(Out1) -> PT1_S16/1
  Product/1 -> PT1_S16/2
  Parameter selection of PT1/2(Out2) -> Product/1
  Constant4/1 -> Switch1/3
  Switch1/1 -> CrCtl_trqDesvHys/1
  stCrCtlOn/1 -> Switch2/2
  Switch/1 -> Switch2/1
  Constant5/1 -> Switch2/3
  Switch2/1 -> Product/2
  PT1_S16/1 -> Switch1/1

== system CrCtl_Governor/Cruise State/CRCTL_SUBGVNR/Governor/Parameter Selection for Ki ==
  CrCtl_stGearRng_mp : Inport
  Constant1 : Constant  Value=CrCtl_KiCruise2IWin_C
  Constant10 : Constant  Value=CrCtl_WinNegCruise1IWin_C
  Constant11 : Constant  Value=CrCtl_WinNegCruise2IWin_C
  Constant12 : Constant  Value=CrCtl_WinNegCruise3IWin_C
  Constant13 : Constant  Value=CrCtl_WinPosCruise1IWin_C
  Constant14 : Constant  Value=CrCtl_WinPosCruise2IWin_C
  Constant15 : Constant  Value=CrCtl_WinPosCruise3IWin_C
  Constant2 : Constant  Value=CrCtl_KiCruise3IWin_C
  Constant3 : Constant  Value=CrCtl_KiPosCruise1IWin_C
  Constant4 : Constant  Value=CrCtl_KiCruise1IWin_C
  Constant5 : Constant  Value=CrCtl_KiPosCruise2IWin_C
  Constant6 : Constant  Value=CrCtl_KiPosCruise3IWin_C
  Constant7 : Constant  Value=CrCtl_KiNegCruise1IWin_C
  Constant8 : Constant  Value=CrCtl_KiNegCruise2IWin_C
  Constant9 : Constant  Value=CrCtl_KiNegCruise3IWin_C
  Multiport Switch{,1..4} (5 alike) : MultiPortSwitch
  Out1 : Outport
  Out2 : Outport  Port=2
  Out3 : Outport  Port=3
  Out4 : Outport  Port=4
  Out5 : Outport  Port=5
  wires:
  Multiport Switch4/1 -> Out5/1
  Multiport Switch3/1 -> Out4/1
  Multiport Switch2/1 -> Out3/1
  Constant11/1 -> Multiport Switch4/3
  Constant12/1 -> Multiport Switch4/4
  Constant10/1 -> Multiport Switch4/2
  Constant14/1 -> Multiport Switch3/3
  Constant15/1 -> Multiport Switch3/4
  Constant13/1 -> Multiport Switch3/2
  Constant8/1 -> Multiport Switch2/3
  Constant9/1 -> Multiport Switch2/4
  Constant7/1 -> Multiport Switch2/2
  Multiport Switch1/1 -> Out2/1
  Constant5/1 -> Multiport Switch1/3
  Constant6/1 -> Multiport Switch1/4
  Constant3/1 -> Multiport Switch1/2
  Multiport Switch/1 -> Out1/1
  Constant2/1 -> Multiport Switch/4
  Constant1/1 -> Multiport Switch/3
  Constant4/1 -> Multiport Switch/2
  CrCtl_stGearRng_mp/1 -> Multiport Switch/1, Multiport Switch1/1, Multiport Switch2/1, Multiport Switch3/1, Multiport Switch4/1

== system CrCtl_Governor/Cruise State/CRCTL_SUBGVNR/Governor/Parameter Selection for Kp ==
  CrCtl_stGearRng_mp : Inport
  Constant1 : Constant  Value=CrCtl_KpCruise2PWin_C
  Constant10 : Constant  Value=CrCtl_WinPosCruise1PWin_C
  Constant11 : Constant  Value=CrCtl_WinPosCruise2PWin_C
  Constant12 : Constant  Value=CrCtl_WinPosCruise3PWin_C
  Constant13 : Constant  Value=CrCtl_WinNegCruise1PWin_C
  Constant14 : Constant  Value=CrCtl_WinNegCruise2PWin_C
  Constant15 : Constant  Value=CrCtl_WinNegCruise3PWin_C
  Constant2 : Constant  Value=CrCtl_KpCruise3PWin_C
  Constant3 : Constant  Value=CrCtl_KpPosCruise1PWin_C
  Constant4 : Constant  Value=CrCtl_KpCruise1PWin_C
  Constant5 : Constant  Value=CrCtl_KpPosCruise2PWin_C
  Constant6 : Constant  Value=CrCtl_KpPosCruise3PWin_C
  Constant7 : Constant  Value=CrCtl_KpNegCruise1PWin_C
  Constant8 : Constant  Value=CrCtl_KpNegCruise2PWin_C
  Constant9 : Constant  Value=CrCtl_KpNegCruise3PWin_C
  Multiport Switch{,1..4} (5 alike) : MultiPortSwitch
  Out1 : Outport
  Out2 : Outport  Port=2
  Out3 : Outport  Port=3
  Out4 : Outport  Port=4
  Out5 : Outport  Port=5
  wires:
  CrCtl_stGearRng_mp/1 -> Multiport Switch4/1, Multiport Switch3/1, Multiport Switch2/1, Multiport Switch1/1, Multiport Switch/1
  Constant4/1 -> Multiport Switch/2
  Constant1/1 -> Multiport Switch/3
  Constant2/1 -> Multiport Switch/4
  Multiport Switch/1 -> Out1/1
  Constant3/1 -> Multiport Switch1/2
  Constant6/1 -> Multiport Switch1/4
  Constant5/1 -> Multiport Switch1/3
  Multiport Switch1/1 -> Out2/1
  Constant7/1 -> Multiport Switch2/2
  Constant9/1 -> Multiport Switch2/4
  Constant8/1 -> Multiport Switch2/3
  Constant10/1 -> Multiport Switch3/2
  Constant12/1 -> Multiport Switch3/4
  Constant11/1 -> Multiport Switch3/3
  Constant13/1 -> Multiport Switch4/2
  Constant15/1 -> Multiport Switch4/4
  Constant14/1 -> Multiport Switch4/3
  Multiport Switch2/1 -> Out3/1
  Multiport Switch3/1 -> Out4/1
  Multiport Switch4/1 -> Out5/1

== system CrCtl_Governor/Deceleration State/CRCTL_SUBRMP/CrCtl_Suspend/Subsystem ==
  PT_trqWhlMinEng : Inport
  CrCtl_trqReqOld : Inport  Port=2
  CrCtl_stSuspAct : Inport  Port=3
  Enable : EnablePort
  Constant5 : Constant  Value=CrCtl_swtSusRmpStp_C
  Constant7 : Constant  Value=CrCtl_facSlpRmp1Sus_C
  Constant8 : Constant  Value=CrCtl_Governor_DT
  RAMP_S16 : CXLib/RAMP_S16
  Relational Operator : RelationalOperator  Operator=~=  OutDataTypeStr=boolean  RndMeth=Simplest
  Switch3 : Switch  Criteria=u2 ~= 0
  s2dt : CXLib/s2dt
  Out : Outport
  Out1 : Outport  Port=2
  wires:
  Constant7/1 -> s2dt/1
  Constant8/1 -> s2dt/2
  s2dt/1 -> RAMP_S16/3, RAMP_S16/2
  CrCtl_stSuspAct/1 -> RAMP_S16/4
  PT_trqWhlMinEng/1 -> Relational Operator/1, Switch3/1, RAMP_S16/1
  Relational Operator/1 -> Out/1
  CrCtl_trqReqOld/1 -> RAMP_S16/5
  Constant5/1 -> Switch3/2
  Switch3/1 -> Relational Operator/2, Out1/1
  RAMP_S16/1 -> Switch3/3

== system CrCtl_Governor/Deceleration State/CRCTL_SUBRMP/CrCtl_Suspend/Subsystem1 ==
  PT_trqWhlMinEng : Inport
  CrCtl_trqReqOld : Inport  Port=2
  AccPed_trqDes : Inport  Port=3
  CrCtl_trqLimAct : Inport  Port=4
  In1 : Inport  Port=5
  In2 : Inport  Port=6
  In3 : Inport  Port=7
  Enable : EnablePort
  Constant10 : Constant  Value=CrCtl_Governor_DT
  Constant6 : Constant  Value=CrCtl_swtSusRmpInit_C
  Constant9 : Constant  Value=CrCtl_facSlpRmp2Sus_C
  MinMax : MinMax  Function=max  Inputs=2
  MinMax1 : MinMax  Function=max  Inputs=2
  RAMP_S1 : CXLib/RAMP_S16
  Relational Operator1 : RelationalOperator  Operator=~=  OutDataTypeStr=boolean  RndMeth=Simplest
  Relational Operator2 : RelationalOperator  Operator=<  OutDataTypeStr=boolean  RndMeth=Simplest
  Relational Operator3 : RelationalOperator  Operator=<  OutDataTypeStr=boolean  RndMeth=Simplest
  Relational Operator4 : RelationalOperator  Operator=<  OutDataTypeStr=boolean  RndMeth=Simplest
  Switch{1..4,6} (5 alike) : Switch  Criteria=u2 ~= 0
  s2dt1 : CXLib/s2dt
  Out1 : Outport
  Out2 : Outport  Port=2
  wires:
  Constant9/1 -> s2dt1/1
  Constant10/1 -> s2dt1/2
  s2dt1/1 -> RAMP_S1/3, RAMP_S1/2
  CrCtl_trqReqOld/1 -> RAMP_S1/1, Relational Operator4/1, Switch6/1, MinMax/1, Relational Operator1/2, Switch2/1, Relational Operator3/1
  Constant6/1 -> Switch3/2
  MinMax/1 -> MinMax1/1
  MinMax1/1 -> Switch4/1, Relational Operator2/1
  CrCtl_trqLimAct/1 -> Switch4/3, Relational Operator2/2
  Relational Operator2/1 -> Switch4/2
  Switch4/1 -> Switch3/1
  AccPed_trqDes/1 -> Relational Operator3/2, MinMax1/2
  PT_trqWhlMinEng/1 -> Switch1/1, Relational Operator4/2, MinMax/2
  Relational Operator4/1 -> Switch1/2
  Switch3/1 -> Switch1/3
  Switch1/1 -> RAMP_S1/5
  In3/1 -> RAMP_S1/4
  In1/1 -> Switch6/2
  In2/1 -> Switch6/3
  Switch6/1 -> Switch3/3
  Relational Operator3/1 -> Switch2/2
  RAMP_S1/1 -> Switch2/3
  Switch2/1 -> Out2/1, Relational Operator1/1
  Relational Operator1/1 -> Out1/1

== system CrCtl_Governor/Deceleration State/CRCTL_SUBRMP/Governor/CrCtl_ARW ==
  CrCtl_swtILimWithP_C : Inport
  CrCtl_trqMin : Inport  Port=2
  CrCtl_trqLimAct : Inport  Port=3
  CrCtl_trqReqPWin_mp : Inport  Port=4
  CrCtl_trqReqIWin_mp : Inport  Port=5
  Add : Sum  Inputs=+-  OutDataTypeStr=Trq_Nm
  Add1 : Sum  Inputs=+-  OutDataTypeStr=Trq_Nm
  Relational Operator : RelationalOperator  Operator=<  OutDataTypeStr=boolean  RndMeth=Simplest
  Relational Operator1 : RelationalOperator  Operator=>  OutDataTypeStr=boolean  RndMeth=Simplest
  Saturation_S1 : CXLib/Saturation_S16
  Saturation_S16 : CXLib/Saturation_S16
  Switch{,1..3} (4 alike) : Switch  Criteria=u2 ~= 0
  CrCtl_stInit_mp : Outport
  Limit : Outport  Port=2
  wires:
  CrCtl_trqMin/1 -> Switch2/3, Relational Operator/2, Add/1, Saturation_S16/2
  CrCtl_trqLimAct/1 -> Switch3/3, Relational Operator1/2, Add1/1, Saturation_S16/3
  CrCtl_trqReqIWin_mp/1 -> Relational Operator1/1, Relational Operator/1, Saturation_S1/1, Saturation_S16/1
  CrCtl_swtILimWithP_C/1 -> Switch1/2, Switch/2
  Switch/1 -> CrCtl_stInit_mp/1
  Saturation_S16/2 -> Switch/3
  CrCtl_trqReqPWin_mp/1 -> Add1/2, Add/2
  Saturation_S1/2 -> Switch/1
  Saturation_S1/1 -> Switch1/1
  Saturation_S16/1 -> Switch1/3
  Switch1/1 -> Limit/1
  Switch2/1 -> Saturation_S1/2
  Switch3/1 -> Saturation_S1/3
  Add/1 -> Switch2/1
  Add1/1 -> Switch3/1
  Relational Operator/1 -> Switch2/2
  Relational Operator1/1 -> Switch3/2

== system CrCtl_Governor/Deceleration State/CRCTL_SUBRMP/Governor/PT1 Filtered Torque ==
  stvHysEngBrkReq : Inport
  vDiffCrCtl : Inport  Port=2
  CrCtl_stGearRng_mp : Inport  Port=3
  stCrCtlOn : Inport  Port=4
  Add : Sum  Inputs=+-
  Constant : Constant
  Constant1 : Constant  Value=CrCtl_swtPT1EngBrk_C
  Constant2 : Constant  Value=CrCtl_vEngBrkOffChkOfs_C
  Constant3 : Constant  Value=CrCtl_vHysEngBrkMode_C
  Constant4 : Constant  Value=0.0  OutDataTypeStr=Inherit: Inherit via back propagation
  Constant5 : Constant  Value=0  OutDataTypeStr=VehSpeed_km_h
  Logical Operator : Logic  Operator=NOT  AllPortsSameDT=off  OutDataTypeStr=boolean
  Logical Operator1 : Logic  Operator=OR  AllPortsSameDT=off  OutDataTypeStr=boolean
  PT1_S16 : CXLib/PT1_S16
  Parameter selection of PT1 : Subsystem
  Product : Product  OutDataTypeStr=Trq_Nm
  Relational Operator : RelationalOperator  Operator===  OutDataTypeStr=boolean  RndMeth=Simplest
  Switch : Switch  Criteria=u2 ~= 0
  Switch1 : Switch  Criteria=u2 ~= 0
  Switch2 : Switch  Criteria=u2 ~= 0
  CrCtl_trqDesvHys : Outport
  wires:
  Constant1/1 -> Relational Operator/1
  Constant/1 -> Relational Operator/2
  stvHysEngBrkReq/1 -> Logical Operator/1
  Relational Operator/1 -> Logical Operator1/1
  Logical Operator/1 -> Logical Operator1/2
  Constant2/1 -> Add/1
  Constant3/1 -> Add/2
  Logical Operator1/1 -> Switch1/2, Switch/2
  Add/1 -> Switch/3
  vDiffCrCtl/1 -> Switch/1
  CrCtl_stGearRng_mp/1 -> Parameter selection of PT1/1(CrCtl_stGearRng_mp)
  Parameter selection of PT1/1(Out1) -> PT1_S16/1
  Product/1 -> PT1_S16/2
  Parameter selection of PT1/2(Out2) -> Product/1
  PT1_S16/1 -> Switch1/1
  Constant4/1 -> Switch1/3
  Switch1/1 -> CrCtl_trqDesvHys/1
  stCrCtlOn/1 -> Switch2/2
  Switch/1 -> Switch2/1
  Constant5/1 -> Switch2/3
  Switch2/1 -> Product/2

== system CrCtl_Governor/Deceleration State/CRCTL_SUBRMP/Governor/Parameter Selection for Ki ==
  CrCtl_stGearRng_mp : Inport
  Constant1 : Constant  Value=CrCtl_KiDecl2IWin_C
  Constant10 : Constant  Value=CrCtl_WinNegDecl1IWin_C
  Constant11 : Constant  Value=CrCtl_WinNegDecl2IWin_C
  Constant12 : Constant  Value=CrCtl_WinNegDecl3IWin_C
  Constant13 : Constant  Value=CrCtl_WinPosDecl1IWin_C
  Constant14 : Constant  Value=CrCtl_WinPosDecl2IWin_C
  Constant15 : Constant  Value=CrCtl_WinPosDecl3IWin_C
  Constant2 : Constant  Value=CrCtl_KiDecl3IWin_C
  Constant3 : Constant  Value=CrCtl_KiPosDecl1IWin_C
  Constant4 : Constant  Value=CrCtl_KiDecl1IWin_C
  Constant5 : Constant  Value=CrCtl_KiPosDecl2IWin_C
  Constant6 : Constant  Value=CrCtl_KiPosDecl3IWin_C
  Constant7 : Constant  Value=CrCtl_KiNegDecl1IWin_C
  Constant8 : Constant  Value=CrCtl_KiNegDecl2IWin_C
  Constant9 : Constant  Value=CrCtl_KiNegDecl3IWin_C
  Multiport Switch{,1..4} (5 alike) : MultiPortSwitch
  Out1 : Outport
  Out2 : Outport  Port=2
  Out3 : Outport  Port=3
  Out4 : Outport  Port=4
  Out5 : Outport  Port=5
  wires:
  Multiport Switch4/1 -> Out5/1
  Multiport Switch3/1 -> Out4/1
  Multiport Switch2/1 -> Out3/1
  Constant11/1 -> Multiport Switch4/3
  Constant12/1 -> Multiport Switch4/4
  Constant10/1 -> Multiport Switch4/2
  Constant14/1 -> Multiport Switch3/3
  Constant15/1 -> Multiport Switch3/4
  Constant13/1 -> Multiport Switch3/2
  Constant8/1 -> Multiport Switch2/3
  Constant9/1 -> Multiport Switch2/4
  Constant7/1 -> Multiport Switch2/2
  Multiport Switch1/1 -> Out2/1
  Constant5/1 -> Multiport Switch1/3
  Constant6/1 -> Multiport Switch1/4
  Constant3/1 -> Multiport Switch1/2
  Multiport Switch/1 -> Out1/1
  Constant2/1 -> Multiport Switch/4
  Constant1/1 -> Multiport Switch/3
  Constant4/1 -> Multiport Switch/2
  CrCtl_stGearRng_mp/1 -> Multiport Switch/1, Multiport Switch1/1, Multiport Switch2/1, Multiport Switch3/1, Multiport Switch4/1

== system CrCtl_Governor/Deceleration State/CRCTL_SUBRMP/Governor/Parameter Selection for Kp ==
  CrCtl_stGearRng_mp : Inport
  Constant1 : Constant  Value=CrCtl_KpDecl2PWin_C
  Constant10 : Constant  Value=CrCtl_WinPosDecl1PWin_C
  Constant11 : Constant  Value=CrCtl_WinPosDecl2PWin_C
  Constant12 : Constant  Value=CrCtl_WinPosDecl3PWin_C
  Constant13 : Constant  Value=CrCtl_WinNegDecl1PWin_C
  Constant14 : Constant  Value=CrCtl_WinNegDecl2PWin_C
  Constant15 : Constant  Value=CrCtl_WinNegDecl3PWin_C
  Constant2 : Constant  Value=CrCtl_KpDecl3PWin_C
  Constant3 : Constant  Value=CrCtl_KpPosDecl1PWin_C
  Constant4 : Constant  Value=CrCtl_KpDecl1PWin_C
  Constant5 : Constant  Value=CrCtl_KpPosDecl2PWin_C
  Constant6 : Constant  Value=CrCtl_KpPosDecl3PWin_C
  Constant7 : Constant  Value=CrCtl_KpNegDecl1PWin_C
  Constant8 : Constant  Value=CrCtl_KpNegDecl2PWin_C
  Constant9 : Constant  Value=CrCtl_KpNegDecl3PWin_C
  Multiport Switch{,1..4} (5 alike) : MultiPortSwitch
  Out1 : Outport
  Out2 : Outport  Port=2
  Out3 : Outport  Port=3
  Out4 : Outport  Port=4
  Out5 : Outport  Port=5
  wires:
  CrCtl_stGearRng_mp/1 -> Multiport Switch4/1, Multiport Switch3/1, Multiport Switch2/1, Multiport Switch1/1, Multiport Switch/1
  Constant4/1 -> Multiport Switch/2
  Constant1/1 -> Multiport Switch/3
  Constant2/1 -> Multiport Switch/4
  Multiport Switch/1 -> Out1/1
  Constant3/1 -> Multiport Switch1/2
  Constant6/1 -> Multiport Switch1/4
  Constant5/1 -> Multiport Switch1/3
  Multiport Switch1/1 -> Out2/1
  Constant7/1 -> Multiport Switch2/2
  Constant9/1 -> Multiport Switch2/4
  Constant8/1 -> Multiport Switch2/3
  Constant10/1 -> Multiport Switch3/2
  Constant12/1 -> Multiport Switch3/4
  Constant11/1 -> Multiport Switch3/3
  Constant13/1 -> Multiport Switch4/2
  Constant15/1 -> Multiport Switch4/4
  Constant14/1 -> Multiport Switch4/3
  Multiport Switch2/1 -> Out3/1
  Multiport Switch3/1 -> Out4/1
  Multiport Switch4/1 -> Out5/1

== system CrCtl_Governor/Resume From Above/CRCTL_SUBRMP/CrCtl_Suspend/Subsystem ==
  PT_trqWhlMinEng : Inport
  CrCtl_trqReqOld : Inport  Port=2
  CrCtl_stSuspAct : Inport  Port=3
  Enable : EnablePort
  Constant5 : Constant  Value=CrCtl_swtSusRmpStp_C
  Constant7 : Constant  Value=CrCtl_facSlpRmp1Sus_C
  Constant8 : Constant  Value=CrCtl_Governor_DT
  RAMP_S16 : CXLib/RAMP_S16
  Relational Operator : RelationalOperator  Operator=~=  OutDataTypeStr=boolean  RndMeth=Simplest
  Switch3 : Switch  Criteria=u2 ~= 0
  s2dt : CXLib/s2dt
  Out : Outport
  Out1 : Outport  Port=2
  wires:
  Constant7/1 -> s2dt/1
  Constant8/1 -> s2dt/2
  s2dt/1 -> RAMP_S16/3, RAMP_S16/2
  CrCtl_stSuspAct/1 -> RAMP_S16/4
  PT_trqWhlMinEng/1 -> Relational Operator/1, Switch3/1, RAMP_S16/1
  Relational Operator/1 -> Out/1
  CrCtl_trqReqOld/1 -> RAMP_S16/5
  Constant5/1 -> Switch3/2
  Switch3/1 -> Relational Operator/2, Out1/1
  RAMP_S16/1 -> Switch3/3
